simulink model "PitchAttitudeHold_Comp"  (R2018b)
settings: Solver=VariableStepAuto  StartTime=0.0  StopTime=20  RelTol=1e-3
libraries: simulink x1
settings Model: Creator=cdjsd  LastModifiedBy=cdjsd

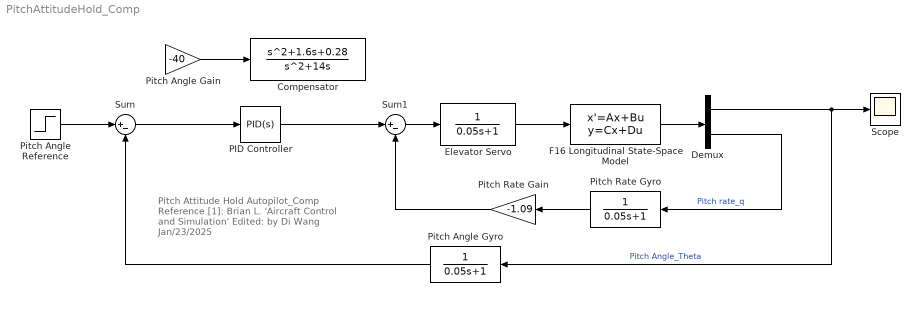
== system PitchAttitudeHold_Comp ==
  note: Pitch Attitude Hold Autopilot_Comp
      | Reference [1]: Brian L. 'Aircraft Control and Simulation'
      | Edited: by Di Wang Jan/23/2025
  Compensator : TransferFcn  Numerator=[1 1.6 0.28]  Denominator=[1 14 0]
  Demux : Demux  Outputs=2
  Elevator Servo : TransferFcn  Denominator=[0.05 1]
  F16 Longitudinal State-Space Model : StateSpace  A=|  B=[0; 0; 0; -0.010992]  C=|  D=[0;0]  InitialCondition=0
      A=|
      | [-3.8916e-2 1.8992e1 -3.2139e1 0;
      |      -1.0285e-3 -6.4537e-1 5.6129e-3 1;
      |      0 0 0 1;
      |      8.0847e-5 -7.7287e-1 -8.0979e-4 -5.29e-1]
      C=|
      | [0 0 57.296 0;
      |      0 0 0 57.296]
  PID Controller : simulink/Continuous/PID Controller  Controller=PID  Form=Parallel  TimeDomain=Continuous-time  SampleTime=-1  IntegratorMethod=Forward Euler  FilterMethod=Forward Euler  ControllerParametersSource=internal  P=-11.2472088416638  I=-4.89388134550719  D=-6.09046644358253  UseFilter=on  N=474.13371150715  TunerSelectOption=Transfer Function Based (PID Tuner App)  InitialConditionSource=internal  InitialConditionForIntegrator=0  InitialConditionForFilter=0  DifferentiatorICPrevScaledInput=0  ExternalReset=none  TrackingMode=off  Kt=1  LimitOutput=off  UpperSaturationLimit=inf  LowerSaturationLimit=-inf  LinearizeAsGain=on  AntiWindupMode=none  Kb=1  POutMin=[]  POutMax=[]  IOutMin=[]  IOutMax=[]  DOutMin=[]  DOutMax=[]  NOutMin=[]  NOutMax=[]  SumOutMin=[]  SumOutMax=[]  SaturationOutMin=[]  SaturationOutMax=[]  PParamMin=[]  PParamMax=[]  IParamMin=[]  IParamMax=[]  DParamMin=[]  DParamMax=[]  NParamMin=[]  NParamMax=[]  KbParamMin=[]  KbParamMax=[]  KtParamMin=[]  KtParamMax=[]  KbOutMin=[]  KbOutMax=[]  KtOutMin=[]  KtOutMax=[]  IntegratorOutMin=[]  IntegratorOutMax=[]  FilterOutMin=[]  FilterOutMax=[]  SumI1OutMin=[]  SumI1OutMax=[]  SumI2OutMin=[]  SumI2OutMax=[]  SumI3OutMin=[]  SumI3OutMax=[]  SumI4OutMin=[]  SumI4OutMax=[]  SumDOutMin=[]  SumDOutMax=[]  DifferentiatorOutMin=[]  DifferentiatorOutMax=[]  FilterDiffOutCoefMin=[]  FilterDiffOutCoefMax=[]  ReciprocalOutMin=[]  ReciprocalOutMax=[]  SumDenOutMin=[]  SumDenOutMax=[]  SumNumOutMin=[]  SumNumOutMax=[]  DivideOutMin=[]  DivideOutMax=[]  IntegratorContinuousStateAttributes=''  IntegratorStateMustResolveToSignalObject=off  IntegratorRTWStateStorageClass=Auto  FilterContinuousStateAttributes=''  FilterStateMustResolveToSignalObject=off  FilterRTWStateStorageClass=Auto  ParallelPVariant=InternalParameters  IdealPVariant=Disabled  IVariant=InternalParameters  DVariant=InternalParameters  IntegratorVariant=Continuous  SatVariant=Disabled  AWVariant=Passthrough  PCopyVariant=Disabled  TRVariant=Disabled  FdbkBlocksVariant=Forward  IdealPFdbkVariant=Disabled  SatFdbkVariant=Disabled  DerivativeFilterVariant=ContFilter  NVariant=InternalParameters  NCopyVariant=Disabled  FilterICVariant=InternalICsFilter  IntegratorICVariant=InternalICs  ExternalResetVariant=Disabled  TRSumVariant=Passthrough  SumFdbkVariant=Disabled  SumVariant=Sum_PID
  Pitch Angle Gain : Gain  Gain=-40
  Pitch Angle Gyro : TransferFcn  Denominator=[0.05 1]
  Pitch Angle Reference : Step  SampleTime=0
  Pitch Rate Gain : Gain  Gain=-1.09
  Pitch Rate Gyro : TransferFcn  Denominator=[0.05 1]
  Scope : Scope
  Sum : Sum  Inputs=|+-
  Sum1 : Sum  Inputs=|+-
  wires:
  Pitch Angle Reference/1 -> Sum/1
  Sum/1 -> PID Controller/1
  PID Controller/1 -> Sum1/1
  F16 Longitudinal State-Space Model/1 -> Demux/1
  Pitch Rate Gyro/1 -> Pitch Rate Gain/1
  Pitch Rate Gain/1 -> Sum1/2
  Elevator Servo/1 -> F16 Longitudinal State-Space Model/1
  Sum1/1 -> Elevator Servo/1
  Pitch Angle Gyro/1 -> Sum/2
  Demux/2 -> Pitch Rate Gyro/1  "Pitch rate_q"
  Demux/1 -> Pitch Angle Gyro/1, Scope/1  "Pitch Angle_Theta"
  Pitch Angle Gain/1 -> Compensator/1
